simulink model "primer_desacople"  (R2020a)
settings: Solver=VariableStepAuto  StartTime=0.0  StopTime=10.0  RelTol=1e-3
model workspace: external: MATLAB File D:\Ferran\Facultad\UNCuyo\Meca\Automática y Máquinas Eléctricas\Proyecto final\matlab2\parametros_y_especs\parametros_y_especif.m (data not in the file)
undefined symbols (not defined in the file): lambda_m, Ld, Lq, Pp
settings Model: Creator=Ferran  LastModifiedBy=Ferran

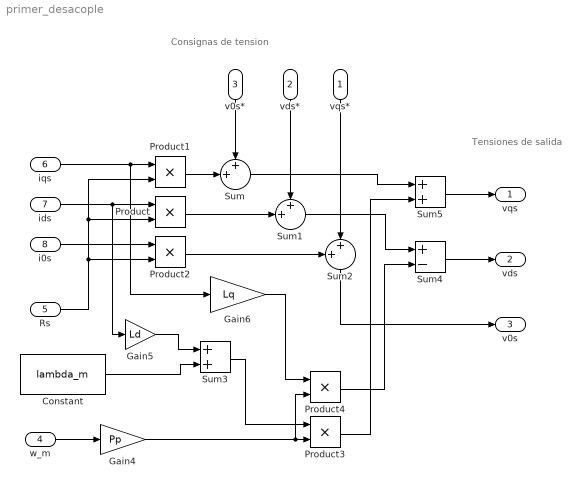
== system primer_desacople ==
  note: Tensiones
      | de salida
  note: Consignas de tension
  vqs* : Inport
  vds* : Inport  Port=2
  v0s* : Inport  Port=3
  w_m : Inport  Port=4
  Rs : Inport  Port=5
  iqs : Inport  Port=6
  ids : Inport  Port=7
  i0s : Inport  Port=8
  Constant : Constant  Value=lambda_m
  Gain4 : Gain  Gain=Pp
  Gain5 : Gain  Gain=Ld
  Gain6 : Gain  Gain=Lq
  Product{,1..4} (5 alike) : Product
  Sum : Sum  Inputs=++|
  Sum1 : Sum  Inputs=++|
  Sum2 : Sum  Inputs=++|
  Sum3 : Sum
  Sum4 : Sum  Inputs=+-
  Sum5 : Sum
  vqs : Outport
  vds : Outport  Port=2
  v0s : Outport  Port=3
  wires:
  Rs/1 -> Product2/2, Product/2, Product1/2
  iqs/1 -> Product1/1, Gain6/1
  ids/1 -> Product/1, Gain5/1
  i0s/1 -> Product2/1
  vds*/1 -> Sum1/1
  vqs*/1 -> Sum2/2
  Product/1 -> Sum1/2
  Product2/1 -> Sum2/1
  w_m/1 -> Gain4/1
  Gain4/1 -> Product4/2, Product3/2
  Constant/1 -> Sum3/2
  Gain5/1 -> Sum3/1
  Sum3/1 -> Product3/1
  Sum2/1 -> v0s/1
  Gain6/1 -> Product4/1
  Product1/1 -> Sum/2
  v0s*/1 -> Sum/1
  Sum/1 -> Sum5/1
  Sum1/1 -> Sum4/1
  Product3/1 -> Sum5/2
  Product4/1 -> Sum4/2
  Sum4/1 -> vds/1
  Sum5/1 -> vqs/1
